simulink model "lib_testValidity"  (R2019a)
settings: Solver=VariableStepAuto  StartTime=0.0  StopTime=tfinal  RelTol=1e-3
model workspace (MAT data in the model file):
  q_init = Simulink.Parameter
  q_init.DataType = 'auto'
  q_init.Dimensions = [0 0]
values from neighbouring files (symbols this model uses):
  Bb = Bb./norm(Bb)    [lib_testValidity_main.m]
  del_t = tspan(2)-tspan(1)    [lib_testValidity_main.m]
  Ri = Ri./norm(Ri)    [lib_testValidity_main.m]
libraries: MEKF_SensorCheck_Lib2018 x1
settings Model: Creator=kylle  LastModifiedBy=kylle
settings SolverCC: ConsecutiveZCsStepRelTol=0.00001
settings DataIOCC: TimeSaveName=timeoutNew  OutputSaveName=youtNew

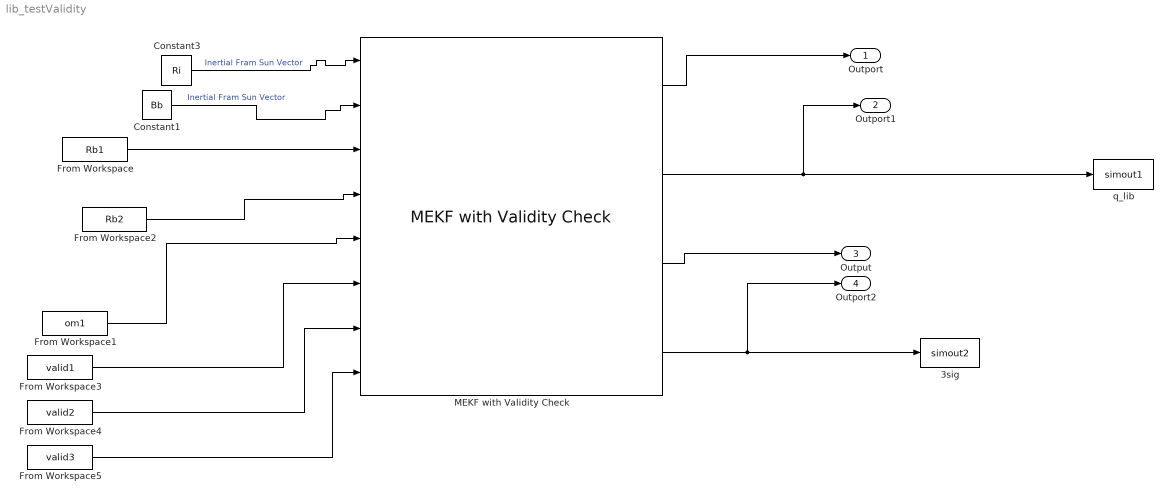
== system lib_testValidity ==
  3sig : ToWorkspace  VariableName=simout2  SaveFormat=Timeseries  SampleTime=-1
  Constant1 : Constant  Value=Bb  VectorParams1D=off
  Constant3 : Constant  Value=Ri  VectorParams1D=off
  From Workspace : FromWorkspace  VariableName=Rb1  SampleTime=del_t
  From Workspace1 : FromWorkspace  VariableName=om1  SampleTime=del_t
  From Workspace2 : FromWorkspace  VariableName=Rb2  SampleTime=del_t
  From Workspace3 : FromWorkspace  VariableName=valid1  SampleTime=del_t
  From Workspace4 : FromWorkspace  VariableName=valid2  SampleTime=del_t
  From Workspace5 : FromWorkspace  VariableName=valid3  SampleTime=del_t
  MEKF with Validity Check : MEKF_SensorCheck_Lib2018/MEKF with Validity Check  SystemSampleTime=-1
  q_lib : ToWorkspace  VariableName=simout1  SaveFormat=Timeseries  SampleTime=-1
  Outport : Outport
  Outport1 : Outport  Port=2
  Output : Outport  Port=3
  Outport2 : Outport  Port=4
  wires:
  From Workspace1/1 -> MEKF with Validity Check/5
  MEKF with Validity Check/3 -> Output/1
  Constant3/1 -> MEKF with Validity Check/1  "Inertial Fram Sun Vector"
  MEKF with Validity Check/1 -> Outport/1
  Constant1/1 -> MEKF with Validity Check/2  "Inertial Fram Sun Vector"
  From Workspace/1 -> MEKF with Validity Check/3
  From Workspace2/1 -> MEKF with Validity Check/4
  From Workspace3/1 -> MEKF with Validity Check/6
  From Workspace4/1 -> MEKF with Validity Check/7
  From Workspace5/1 -> MEKF with Validity Check/8
  MEKF with Validity Check/2 -> q_lib/1, Outport1/1
  MEKF with Validity Check/4 -> 3sig/1, Outport2/1
